simulink model "TVLQR_w_pss"  (R2024b)
settings: Solver=FixedStepDiscrete  StartTime=0.0  StopTime=11380*50  FixedStep=1  RelTol=1e-3
values from neighbouring files (symbols this model uses):
  Ad = sys_d.A    [TVLQR_dist.m]
  Bd = sys_d.B    [TVLQR_dist.m]
  Cd = sys_d.C    [TVLQR_dist.m]
  Dd = sys_d.D    [TVLQR_dist.m]
  Pss = care(A, L, Q, eye(6))    [TVLQR_dist.m]
  R_inv = diag(1./diag(R))    [TVLQR_dist.m]
settings Model: Creator=zalak  LastModifiedBy=zalak

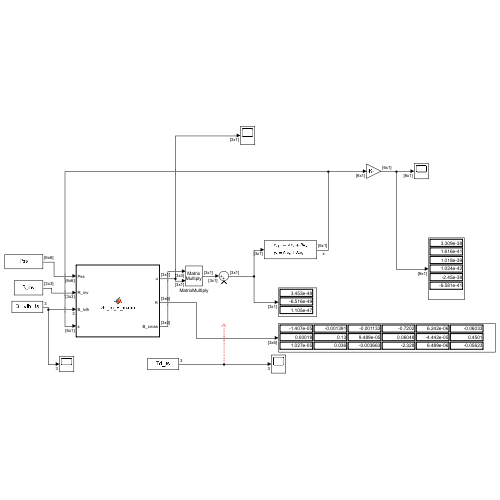
[thumbnail: Simulink's stored preview of the top-level diagram]
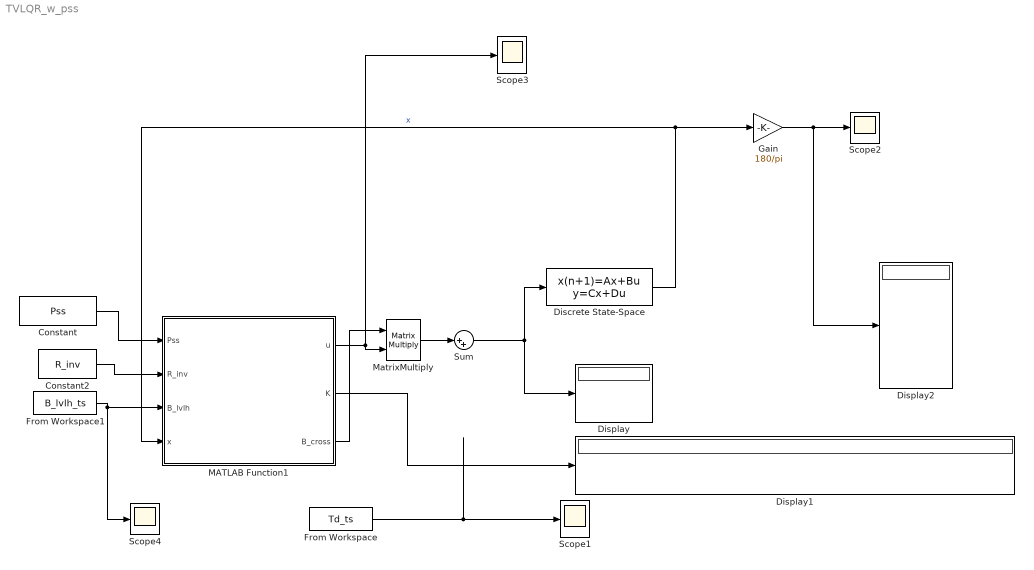
== system TVLQR_w_pss ==
  Constant : Constant  Value=Pss
  Constant2 : Constant  Value=R_inv
  Discrete State-Space : DiscreteStateSpace  A=Ad  B=Bd  C=Cd  D=Dd  InitialCondition=[20*pi/180;0;0;0;0;0]
  Display : Display
  Display1 : Display
  Display2 : Display
  From Workspace : FromWorkspace  VariableName=Td_ts
  From Workspace1 : FromWorkspace  VariableName=B_lvlh_ts  SampleTime=1
  Gain : Gain  Gain=180/pi
  MATLAB Function1 : MATLAB Function  TreatAsAtomicUnit=on
  MatrixMultiply : Product  Multiplication=Matrix(*)
  Scope{1..4} (4 alike) : Scope
  Sum : Sum  Inputs=|++
  wires:
  Gain/1 -> Display2/1, Scope2/1
  From Workspace1/1 -> MATLAB Function1/3(B_lvlh), Scope4/1
  Constant2/1 -> MATLAB Function1/2(R_inv)
  MATLAB Function1/2(K) -> Display1/1
  MATLAB Function1/1(u) -> Scope3/1, MatrixMultiply/2
  Discrete State-Space/1 -> Gain/1, MATLAB Function1/4(x)  "x"
  MATLAB Function1/3(B_cross) -> MatrixMultiply/1
  MatrixMultiply/1 -> Sum/1
  From Workspace/1 -> Scope1/1
  Sum/1 -> Discrete State-Space/1, Display/1
  Constant/1 -> MATLAB Function1/1(Pss)

== matlab function TVLQR_w_pss/MATLAB Function1 ==
  data: Pss input; R_inv input; B_lvlh input; x input; u output; K output; B_cross output
function [u, K, B_cross] = lvlh_to_K_matrix( Pss, R_inv, B_lvlh, x)
% TVLQR step — dipole-based magnetorquer control
%
%   u (3x1)   commanded magnetic dipole moment [A·m²]
%   K (3x6)   instantaneous LQR gain
%   P_next    Riccati state to feed back next step
%
% State convention (matches the A used in setup):
%   x = [phi, p, psi, r, theta, q]'
%       roll, roll-rate, yaw, yaw-rate, pitch, pitch-rate
% GOOSE 2U inertia [kg·m²]
mass = 2.0;  Lx = 0.226;  Ly = 0.100;  Lz = 0.100;
Ix = (1/12)*mass*(Ly^2+Lz^2);   % = 0.00333
Iy = (1/12)*mass*(Lx^2+Lz^2);   % = 0.01020
Iz = (1/12)*mass*(Lx^2+Ly^2);   % = 0.01020
m_max = 0.2;

%% Step 1 — Euler angles in the correct slots
phi   = x(1);
theta = x(3);
psi   = x(5);
Rx = [1,         0,          0;
      0,  cos(phi),  sin(phi);
      0, -sin(phi),  cos(phi)];
Ry = [cos(theta), 0, -sin(theta);
              0,  1,           0;
      sin(theta), 0,  cos(theta)];
Rz = [ cos(psi), sin(psi), 0;
      -sin(psi), cos(psi), 0;
              0,        0, 1];
R_lvlh2body = Rz * Ry * Rx;
B_body      = R_lvlh2body * B_lvlh(:);
%% Step 2 — Build instantaneous input matrix B_tv
% Magnetorquer:  T = m × B = -[B×] m  →  call -[B×] = B_cross
Bx = B_body(1);  By = B_body(2);  Bz = B_body(3);
B_cross = [   0,   Bz,  -By;
            -Bz,    0,   Bx;
             By,  -Bx,    0 ];
B_tv = zeros(6,3);
B_tv(2,:) = B_cross(1,:) / Ix;   % Tx → p
B_tv(4,:) = B_cross(2,:) / Iy;   % Ty → q
B_tv(6,:) = B_cross(3,:) / Iz;   % Tz → r
%% Step 4 — Gain and control law
K = -3.5575 * R_inv * (B_tv' * Pss);
u_nom = K * x;          % dipole command [A·m²] — note the minus sign
%% Step 5 — Saturate at hardware limit (per axis)
beta = max(abs(u_nom) / m_max);
u = u_nom / max(beta, 1);
end
